simulink model "Lab1_parameter_estimation_student"  (R2025b)
settings: Solver=FixedStepAuto  StartTime=0.0  StopTime=18  FixedStep=0.0001  RelTol=1e-3
values from neighbouring files (symbols this model uses):
  motor_B = 1    [Lab1_motor_params_student.m]    (also in loadEstimatedValue.m = Estimated_data(i).Value)
  motor_Eff = 0.5    [Lab1_motor_params_student.m]    (also in loadEstimatedValue.m = Estimated_data(i).Value)
  motor_J = 1    [Lab1_motor_params_student.m]    (also in loadEstimatedValue.m = Estimated_data(i).Value)
  motor_Ke = 0.05    [Lab1_motor_params_student.m]    (also in loadEstimatedValue.m = Estimated_data(i).Value)
  motor_L = 36.22e-3    (= 0.03622)    [Lab1_motor_params_student.m]    (also in loadEstimatedValue.m = 36.22)
  motor_R = 2.97    [Lab1_motor_params_student.m]    (also in loadEstimatedValue.m)
libraries: simulink x2, eeStairGenerator x1
settings Model: Creator=tanawatp  LastModifiedBy=Asus
settings DataIOCC: OutputOption=AdditionalOutputTimes  OutputTimes=SDO_OutputTimes  ReturnWorkspaceOutputsName=SDOSimTest_Log
settings RTWCC: GPUComputeCapability=3.5

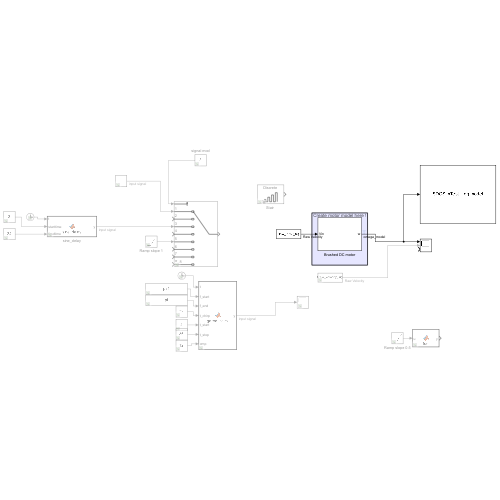
[thumbnail: Simulink's stored preview of the top-level diagram]
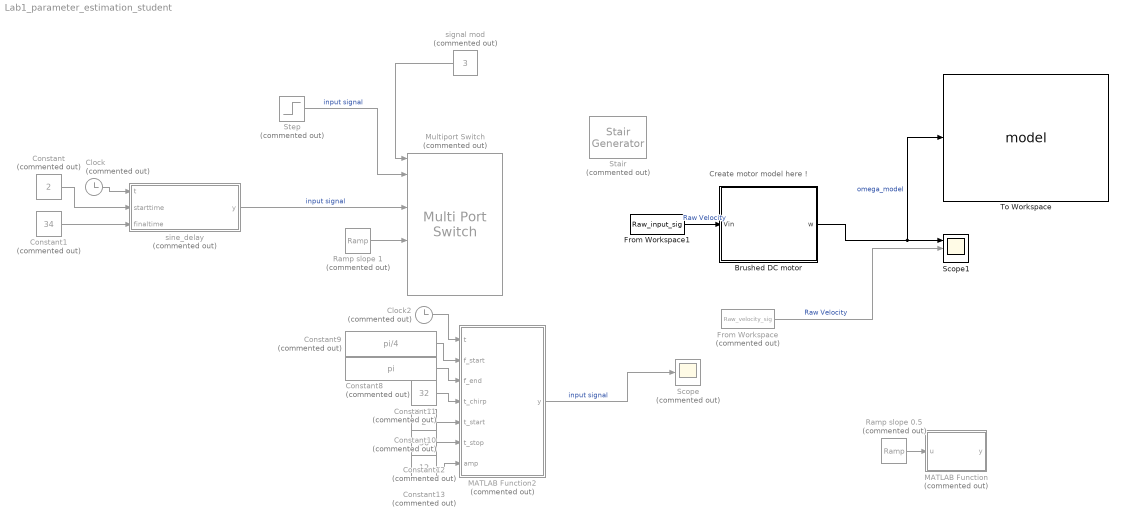
== system Lab1_parameter_estimation_student ==
  note: Create motor model here !
  Brushed DC motor : Subsystem
  Clock : Clock  Commented=on
  Clock2 : Clock  Commented=on
  Constant : Constant  Commented=on  Value=2
  Constant1 : Constant  Commented=on  Value=34
  Constant10 : Constant  Commented=on  Value=2
  Constant11 : Constant  Commented=on  Value=32
  Constant12 : Constant  Commented=on  Value=36
  Constant13 : Constant  Commented=on  Value=12
  Constant8 : Constant  Commented=on  Value=pi
  Constant9 : Constant  Commented=on  Value=pi/4
  From Workspace : FromWorkspace  Commented=on  VariableName=Raw_velocity_sig  SampleTime=0.001
  From Workspace1 : FromWorkspace  VariableName=Raw_input_sig  SampleTime=0.001
  MATLAB Function : MATLAB Function  Commented=on  TreatAsAtomicUnit=on
  MATLAB Function2 : MATLAB Function  Commented=on  TreatAsAtomicUnit=on
  Multiport Switch : MultiPortSwitch  Commented=on  Inputs=8  SaturateOnIntegerOverflow=off  InputSameDT=off
  Ramp slope 0.5 : simulink/Sources/Ramp  Commented=on  slope=1  start=2  InitialOutput=0
  Ramp slope 1 : simulink/Sources/Ramp  Commented=on  slope=1  start=2  InitialOutput=0
  Scope : Scope  Commented=on
      settings: ActiveDisplayYMinimum=-5.6577266323929107  ActiveDisplayYMaximum=3.5509721245815173
  Scope1 : Scope  NumInputPorts=3
      settings: ActiveDisplayYMinimum=-314.92292935859189  ActiveDisplayYMaximum=299.00576613480359
  "Stair " : eeStairGenerator/Stair Generator  Commented=on  LabelModeActiveChoice=Discrete  TimeInput=[2 4 6 8 10 12 14 16]  AmplitudeInput=[3 0 6 0 9 0 12 0]  SampleTime=0.001  RepeatPattern=off  OutDataTypeStr=double
      settings: LibrarySourceBlock=ee_sl_lib/General Control/Stair Generator
  Step : Step  Commented=on  Time=2  After=12  SampleTime=0
  To Workspace : ToWorkspace  VariableName=model  SaveFormat=Timeseries  SampleTime=0.001
  signal mod : Constant  Commented=on  Value=3
  sine_delay : MATLAB Function  Commented=on  TreatAsAtomicUnit=on
  wires:
  Clock/1 -> sine_delay/1(t)
  Constant/1 -> sine_delay/2(starttime)
  Constant1/1 -> sine_delay/3(finaltime)
  Clock2/1 -> MATLAB Function2/1(t)
  Constant9/1 -> MATLAB Function2/2(f_start)
  Constant8/1 -> MATLAB Function2/3(f_end)
  Constant11/1 -> MATLAB Function2/4(t_chirp)
  Constant10/1 -> MATLAB Function2/5(t_start)
  Constant12/1 -> MATLAB Function2/6(t_stop)
  Constant13/1 -> MATLAB Function2/7(amp)
  Ramp slope 0.5/1 -> MATLAB Function/1(u)
  Brushed DC motor/1(w) -> Scope1/1, To Workspace/1  "omega_model"
  From Workspace/1 -> Scope1/2  "Raw Velocity"
  signal mod/1 -> Multiport Switch/1
  Step/1 -> Multiport Switch/2  "input signal"
  sine_delay/1(y) -> Multiport Switch/4  "input signal"
  Ramp slope 1/1 -> Multiport Switch/6
  MATLAB Function2/1(y) -> Scope/1  "input signal"
  From Workspace1/1 -> Brushed DC motor/1(Vin)  "Raw Velocity"

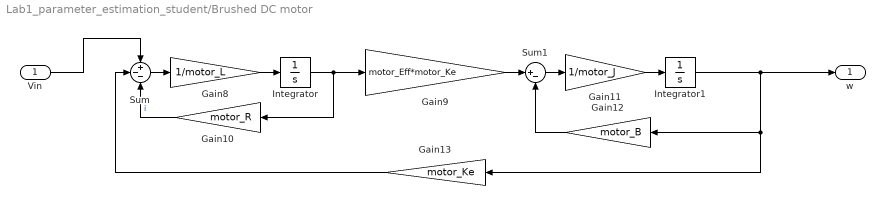
== system Lab1_parameter_estimation_student/Brushed DC motor ==
  Vin : Inport
  Gain10 : Gain  Gain=motor_R
  Gain11 : Gain  Gain=1/motor_J
  Gain12 : Gain  Gain=motor_B
  Gain13 : Gain  Gain=motor_Ke
  Gain8 : Gain  Gain=1/motor_L
  Gain9 : Gain  Gain=motor_Eff*motor_Ke
  Integrator : Integrator
  Integrator1 : Integrator
  Sum : Sum  Inputs=+--
  Sum1 : Sum  Inputs=|+-
  w : Outport
  wires:
  Sum/1 -> Gain8/1
  Gain8/1 -> Integrator/1
  Integrator/1 -> Gain10/1, Gain9/1
  Gain9/1 -> Sum1/1
  Sum1/1 -> Gain11/1
  Gain11/1 -> Integrator1/1
  Gain10/1 -> Sum/3  "i"
  Gain12/1 -> Sum1/2
  Vin/1 -> Sum/1
  Gain13/1 -> Sum/2
  Integrator1/1 -> Gain13/1, Gain12/1, w/1

== matlab function Lab1_parameter_estimation_student/sine_delay ==
  data: t input; y output; starttime input; finaltime input
function y = sine_delay(t, starttime, finaltime)

Amplitude = 12;
Freq = pi/4;

if starttime < t && t < finaltime
    y = sin((t - starttime) * Freq) * Amplitude; 
elseif t >= finaltime
    y = sin((finaltime- starttime) * Freq) * Amplitude; 
else
    y=0;
end

== matlab function Lab1_parameter_estimation_student/MATLAB Function ==
  data: u input; y output
function y = fcn(u)


if u > 12
    y = 12;
else
    y = u;
end

== matlab function Lab1_parameter_estimation_student/MATLAB Function2 ==
  data: t input; y output; f_start input; f_end input; t_chirp input; t_start input; t_stop input; amp input
function y = gated_chirp(t, f_start, f_end, t_chirp, ...
                          t_start, t_stop, amp)
% t        : เวลาปัจจุบัน (วินาที)
% f_start  : ความถี่เริ่มต้น (Hz)
% f_end    : ความถี่สุดท้าย (Hz)
% t_chirp  : ระยะเวลา chirp (วินาที)
% t_start  : เวลาเริ่มสร้างสัญญาณ (วินาที)
% t_stop   : เวลาหยุดสัญญาณ (วินาที)
% amp      : แอมพลิจูด

y = 0;  % ค่าเริ่มต้นนอกช่วงเวลา

if (t >= t_start) && (t <= t_stop)

    % เวลาอ้างอิงภายใน chirp
    tau = t - t_start;

    % จำกัดไม่ให้เกินช่วง chirp
    if tau <= t_chirp
        % linear chirp
        k = (f_end - f_start) / t_chirp;   % sweep rate
        phase = ( f_start*tau + 0.5*k*tau^2 );
        y = amp * sin(phase);
    else
        y = 0;
    end
end
end
